simulink model "Super3_tmp"  (Simulink 8.3)
settings: Solver=ode45  StartTime=0.0  StopTime=10.0  RelTol=1e-3
settings Model: Creator=scaife  LastModifiedBy=bourbouh  CovSFcnEnable=on  ExtModeAutoUpdateStatusClock=off
settings DataIOCC: SignalLoggingName=sigsOut
settings DebuggingCC: SaveWithParameterizedLinksMsg=none  SignalResolutionControl=TryResolveAllWithWarning  SolverPrmCheckMsg=none  MultiTaskDSMMsg=warning  MultiTaskCondExecSysMsg=none  FrameProcessingCompatibilityMsg=error  StateNameClashWarn=none
settings HardwareCC: TargetUnknown=on
settings SFSimCC: SimParseCustomCode=off
settings GRTTargetCC: GeneratePreprocessorConditionals=Use local settings

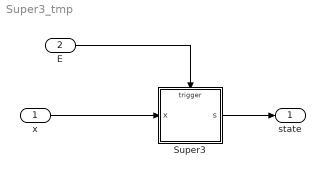
== system Super3_tmp ==
  x : Inport
  E : Inport  Port=2
  Super3 : Stateflow chart  TreatAsAtomicUnit=on
      settings: PermitHierarchicalResolution=ParametersOnly
  state : Outport
  wires:
  E/1 -> Super3/Trigger
  x/1 -> Super3/1(x)
  Super3/1(s) -> state/1

== stateflow chart Super3 ==
  state A
    en : s = 2
  state C
    en : s = 5
  state B
    state B1
      en : s = 4
    state B2
      en : s = 3
    B2 -> B : E[x==3||x==4]
    (junction 9) -> B2 [order 2] : E[x==3]
    B1 -> (junction 9) [order 2] : E[x<=3]
    (junction 10) -> B2 [order 2] : [x==4]
    B1 -> (junction 10) [order 3] : E[x>3]
    (default) -> B1
  state D
    en : s = 1
  B -> C : E[x==0]
  D -> B [order 1] : E[x==0]
  (junction 9) -> D [order 1] : E[x==1]
  D -> A [order 2] : E[x==1]
  (junction 20) -> D [order 2] : [x==0]
  (junction 10) -> C [order 1] : [x==5]
  (junction 20) -> B1 [order 1] : [x>0]
  A -> (junction 20) : E
  C -> A : E[x==0||x==5]
  B1 -> A [order 1] : E[x==2]
  (default) -> A
  data: x input int32; s output double
  events: E input EITHER_EDGE_EVENT
